simulink model "newboostonverter"  (Simulink 8.1)
settings: Solver=ode45  StartTime=0.0  StopTime=.01  RelTol=1e-3
libraries: powerlib x10
settings Model: Creator=USER  LastModifiedBy=KARIKALAN
settings DebuggingCC: StrictBusMsg=Warning

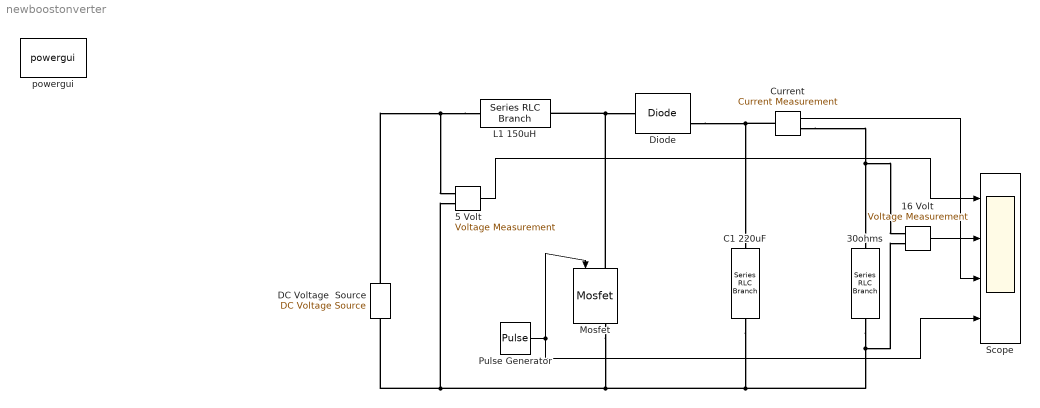
== system newboostonverter ==
  16 Volt : powerlib/Measurements/Voltage Measurement  PhasorSimulation=off  OutputType=Complex  PSBequivalent=0
  30ohms : powerlib/Elements/Series RLC Branch  LConnTagsString=__new0  RConnTagsString=__new0  BranchType=R  Resistance=30  Inductance=1e-3  SetiL0=off  InitialCurrent=0  Capacitance=1e-6  Setx0=off  InitialVoltage=0  Measurements=None
  "5 Volt " : powerlib/Measurements/Voltage Measurement  PhasorSimulation=off  OutputType=Complex  PSBequivalent=0
  C1 220uF : powerlib/Elements/Series RLC Branch  LConnTagsString=__new0  RConnTagsString=__new0  BranchType=C  Resistance=1  Inductance=1e-3  SetiL0=off  InitialCurrent=0  Capacitance=220e-6  Setx0=off  InitialVoltage=0  Measurements=None
  "Current " : powerlib/Measurements/Current Measurement  PhasorSimulation=off  OutputType=Complex  PSBequivalent=0
  DC Voltage  Source : powerlib/Electrical Sources/DC Voltage Source  Amplitude=5  Measurements=None
  Diode : powerlib/Power Electronics/Diode  Ron=0.001  Lon=0  Vf=0.8  IC=0  UseSnubber=off  Rs=500  Cs=250e-9  Measurements=on
  L1 150uH : powerlib/Elements/Series RLC Branch  LConnTagsString=__new0  RConnTagsString=__new0  BranchType=L  Resistance=1  Inductance=150e-6  SetiL0=off  InitialCurrent=0  Capacitance=220e-6  Setx0=off  InitialVoltage=0  Measurements=None
  Mosfet : powerlib/Power Electronics/Mosfet  Ron=0.1  Lon=0  Rd=0.01  Vfd=0  IC=0  Rs=1e5  Cs=inf  Measurements=on
  Pulse Generator : DiscretePulseGenerator  PulseType=Time based  Amplitude=3  Period=4e-5  PulseWidth=66.67
  Scope : Scope  NumInputPorts=4
      settings: TickLabels=on  ShowLegends=on  YMin=0~0~0~-5  YMax=10~50~5~10
  powergui : powerlib/powergui  Priority=1  SimulationMode=Continuous  SolverType=Tustin  SampleTime=50e-6  frequency=60  SPID=off  DisableSnubberDevices=off  DisableRonSwitches=off  DisableVfSwitches=off  SwTol=0  Interpol=off  DisplayEquations=off  frequencyindice=0  Pbase=100e6  ErrMax=1e-4  Iterations=50  UnitsV=kV  UnitsW=MW  FunctionMessages=off  echomessages=off  HookPort=off  EnableUseOfTLC=off  x0status=blocks  RestoreLinks=warning  ResistiveCurrentMeasurement=off  Frange=[0:2:500]  Ylog=off  Xlog=on  ShowGrid=off  save=off  variable=ZData  ZoomFFT=on  StartTime=0.0  cycles=1  DisplayStyle=1  fundamental=60  FreqAxis=off  MaxFrequency=1000  frequencyindicesteady=1  RmsSteady=1  display=off  Ts=0  methode=off
  wires:
  "5 Volt "/1 -> Scope/1
  16 Volt/1 -> Scope/2
  "Current "/1 -> Scope/3
  Pulse Generator/1 -> Mosfet/1, Scope/4
  connections:
  L1 150uH/RConn1 -- DC Voltage  Source/RConn1 -- "5 Volt "/LConn1
  Mosfet/LConn1 -- L1 150uH/LConn1 -- Diode/LConn1
  "Current "/LConn1 -- C1 220uF/LConn1 -- Diode/RConn1
  "Current "/RConn1 -- 30ohms/LConn1 -- 16 Volt/LConn1
  Mosfet/RConn1 -- C1 220uF/RConn1 -- 30ohms/RConn1 -- 16 Volt/LConn2 -- DC Voltage  Source/LConn1 -- "5 Volt "/LConn2
